simulink model "TVModel"  (R2022a)
settings: Solver=FixedStepDiscrete  StartTime=0.0  StopTime=10.0  FixedStep=0.02  MaxStep=0.01  RelTol=1e-3
undefined symbols (not defined in the file or in its folder): MB, TV, TV_OLD
libraries: simulink x22, simulink_extras x14, slpidlib x8, fuzblock x5, controlLib x4, dspstat3 x4, eeGeneralControl x3, cstblocks x3, eeSlidingModeController x1, sharedTrackingLibrary x1
(part 8 of 8)

== stateflow chart TVModel/Subsystem/Subsystem1/Torque Distribution/MPC/Faults Detection/Overlap Chart ==
  state Stop
    en:
    torque_flag = 0;
  state Go
    en:
    torque_flag = 1;
  (default) -> Go
  Go -> Stop : [brake > 0]
  Stop -> Go : [(brake<=0.05 && throttle<0.05)]
  data: throttle input; brake input; torque_flag output

== matlab function TVModel/Subsystem/Subsystem1/Torque Distribution/MPC/Mz Generation/MATLAB Function2 ==
  data: Nhorizon input; vx input; vy input; Nx output; YRD input; r input; delta input; ax input; ay input; kappa input
function Nx =fcn(Nhorizon,vx,vy,YRD,r,delta,ax,ay,kappa)

g   = 9.81;            % [m/s^2]                          
wd  = 0.48;             % [~]         
wb  = 1.53;            % [~]          
tf  = 1.27;            % [m]          
tr  = 1.27;            % [m]          
m   = 195+75;          % [Kg]            
Iz  = 180;             % [Kg*m^2]      % 227    
a   = wb*wd;           % [m]            
b   = wb - a;          % [m]            
hcog = 0.29;           % [m]           
Fzf  = m*g/2*(wd);     % [N]                 
Fzr  = m*g/2*(1-wd);   % [N]                   
tau = 13.5;            % [~]          
rs  = 0.235;           % [m]     
LMU = 0.8;
dt = 0.02;

% ~~~~~~~~~~~~~~~~~~~~~~~~~~~ Aero parameters ~~~~~~~~~~~~~~~~~~~~~~~~~~~~~
xcop = 0.6810;
hcop = 0.576;          % [m]      
rho = 1.225;           % [Kg/m^3]     
CdA = 1.708;           % [m]     
ClA = 5.14;            % [m]   

kappa_FL = kappa(1);
kappa_FR = kappa(2);
kappa_RL = kappa(3);
kappa_RR = kappa(4);

% ~~~~~~~~~~~~~~~~~~~~~~~~~~~ Aerodynamics ~~~~~~~~~~~~~~~~~~~~~~~~~~~~~~~~
Faerox = 0.5*rho*CdA*vx^2;
Faeroz = 0.5*rho*ClA*vx^2;

% ~~~~~~~~~~~~~~~~~~~~~~~~~~~ Slip Angles ~~~~~~~~~~~~~~~~~~~~~~~~~~~~~~~~~
alpha_FL =  (atan((vy + r*a)./(vx - r*tf/2)) - delta);
alpha_FR =  (atan((vy + r*a)./(vx + r*tf/2)) - delta);
alpha_RL =  (atan((vy - r*b)./(vx - r*tr/2)));     
alpha_RR =  (atan((vy - r*b)./(vx + r*tr/2)));     

% ~~~~~~~~~~~~~~~~~~~~~~~~~~~ Vertical loads ~~~~~~~~~~~~~~~~~~~~~~~~~~~~~~

Fz_FL = Fzf - 0.5*(m/tf*hcog).*ay + 0.5*Faeroz*(1-xcop/wb) - 0.5*Faerox/wb*hcop - 0.5*(m/wb*hcog).*ax;
Fz_FR = Fzf + 0.5*(m/tf*hcog).*ay + 0.5*Faeroz*(1-xcop/wb) - 0.5*Faerox/wb*hcop - 0.5*(m/wb*hcog).*ax;
Fz_RL = Fzr - 0.5*(m/tr*hcog).*ay + 0.5*Faeroz*(xcop/wb) + 0.5*Faerox/wb*hcop + 0.5*(m/wb*hcog).*ax;
Fz_RR = Fzr + 0.5*(m/tr*hcog).*ay + 0.5*Faeroz*(xcop/wb) + 0.5*Faerox/wb*hcop + 0.5*(m/wb*hcog).*ax;

% ~~~~~~~~~~~~~~~~~~~~~~~~ Camber gain with steer ~~~~~~~~~~~~~~~~~~~~~~~~~
% ~~~~~~~~~~~~~~~~~~~~~~~~~~ Lateral forces ~~~~~~~~~~~~~~~~~~~~~~~~~~~~~~~
Fy_FL = tire_model(Fz_FL,kappa_FL,alpha_FL,0,LMU);
Fy_FR = tire_model(Fz_FR,kappa_FR,alpha_FR,0,LMU);
Fy_RL = tire_model(Fz_RL,kappa_RL,alpha_RL,0,LMU);
Fy_RR = tire_model(Fz_RR,kappa_RR,alpha_RR,0,LMU);

% ~~~~~~~~~~~~~~~~~~~~~~~~~~~ E.o.M. Balance ~~~~~~~~~~~~~~~~~~~~~~~~~~~~~~
Ny = (Fy_FL + Fy_FR).*cos(delta).*a - b*(Fy_RL + Fy_RR) + tf*(- (Fy_FR - Fy_FL).*sin(delta))/2;
% ~~~~~~~~~~~~~~~~~~~~~~~~~~~ System Dynamics f(x,u) ~~~~~~~~~~~~~~~~~~~~~~     
Nx = (YRD-r)/(dt*Nhorizon)*Iz - Ny;

if(isnan(Nx))
    Nx = 0;
end
end
%% ~~~~~~~~~~~~~~~~~~~~~~~~~~ Functions ~~~~~~~~~~~~~~~~~~~~~~~~~~~~~~~~~~~
function y = tire_model(Fz,kappa,alpha,gamma,LMU)
% Old tir file
% y = - (1.0*cos(0.958*atan((13.9*(3.86e-7*Fz - 1.0*kappa + 2.05e-4))/((12.4*alpha - 0.512)^2 + 1.0)^(1/2) + (atan((13.9*(3.86e-7*Fz - 1.0*kappa + 2.05e-4))/((12.4*alpha - 0.512)^2 + 1.0)^(1/2)) - (13.9*(3.86e-7*Fz - 1.0*kappa + 2.05e-4))/((12.4*alpha - 0.512)^2 + 1.0)^(1/2))*(0.0013*Fz - 2.33)))*(Fz*LMU*(2.59e-6*Fz + 0.0594) - 1.0*Fz*LMU*sin(1.1*atan((1.18*sign(3.32e-6*Fz - 1.0*alpha + 2.0e-5) + 1.0)*(atan((3.41e+4*sin(2.0*atan(8.72e-4*Fz))*(3.32e-6*Fz - 1.0*alpha + 2.0e-5))/(1.1*Fz*LMU*(4.11e-4*Fz - 2.12) - 0.01)) - (3.41e+4*sin(2.0*atan(8.72e-4*Fz))*(3.32e-6*Fz - 1.0*alpha + 2.0e-5))/(1.1*Fz*LMU*(4.11e-4*Fz - 2.12) - 0.01))*(6.75e-4*Fz - 0.451) + (3.41e+4*sin(2.0*atan(8.72e-4*Fz))*(3.32e-6*Fz - 1.0*alpha + 2.0e-5))/(1.1*Fz*LMU*(4.11e-4*Fz - 2.12) - 0.01)))*(4.11e-4*Fz - 2.12)))/cos(0.958*atan((atan((13.9*(3.86e-7*Fz + 2.05e-4))/((12.4*alpha - 0.512)^2 + 1.0)^(1/2)) - (13.9*(3.86e-7*Fz + 2.05e-4))/((12.4*alpha - 0.512)^2 + 1.0)^(1/2))*(0.0013*Fz - 2.33) + (13.9*(3.86e-7*Fz + 2.05e-4))/((12.4*alpha - 0.512)^2 + 1.0)^(1/2))) - (1.0*Fz*LMU*sin(1.94*atan(16.1*kappa))*(1.03e-5*Fz - 2.88e-4)*(4.11e-4*Fz - 2.12))/(225.0*alpha^2 + 1.0)^(1/2);
% New tir file
y = (cos(0.958*atan((13.9*(3.86e-7*Fz - 1.0*kappa + 2.05e-4))/((12.4*alpha - 0.512)^2 + 1.0)^(1/2) + (atan((13.9*(3.86e-7*Fz - 1.0*kappa + 2.05e-4))/((12.4*alpha - 0.512)^2 + 1.0)^(1/2)) - (13.9*(3.86e-7*Fz - 1.0*kappa + 2.05e-4))/((12.4*alpha - 0.512)^2 + 1.0)^(1/2))*(0.0013*Fz - 2.33)))*(Fz*LMU*(7.1e-5*Fz - 0.149) + Fz*LMU*sin(1.34*atan((3.45e+4*sin(2.0*atan(5.59e-4*Fz))*(1.14e-6*Fz - 1.0*alpha + 0.00239))/(1.34*Fz*LMU*(2.82e-4*Fz - 2.02) - 0.01) - 1.0*(0.26*sign(1.14e-6*Fz - 1.0*alpha + 0.00239) + 1.0)*(3.99e-5*Fz - 0.521)*(atan((3.45e+4*sin(2.0*atan(5.59e-4*Fz))*(1.14e-6*Fz - 1.0*alpha + 0.00239))/(1.34*Fz*LMU*(2.82e-4*Fz - 2.02) - 0.01)) - (3.45e+4*sin(2.0*atan(5.59e-4*Fz))*(1.14e-6*Fz - 1.0*alpha + 0.00239))/(1.34*Fz*LMU*(2.82e-4*Fz - 2.02) - 0.01))))*(2.82e-4*Fz - 2.02)))/cos(0.958*atan((atan((13.9*(3.86e-7*Fz + 2.05e-4))/((12.4*alpha - 0.512)^2 + 1.0)^(1/2)) - (13.9*(3.86e-7*Fz + 2.05e-4))/((12.4*alpha - 0.512)^2 + 1.0)^(1/2))*(0.0013*Fz - 2.33) + (13.9*(3.86e-7*Fz + 2.05e-4))/((12.4*alpha - 0.512)^2 + 1.0)^(1/2))) - (1.0*Fz*LMU*sin(1.94*atan(16.1*kappa))*(2.82e-4*Fz - 2.02)*(1.03e-5*Fz - 2.88e-4))/(225.0*alpha^2 + 1.0)^(1/2);
end

== matlab function TVModel/Subsystem/Subsystem1/Torque Distribution/MPC/States Constraints/Cross Check ==
  data: ubx_in input; bounds input; ubx_out output; lbx_in input; lbx_out output; epsilon input; throttle input; brake input
function [ubx_out,lbx_out] = fcn(ubx_in,bounds,lbx_in,epsilon,throttle,brake)
    
    ubx_out = ubx_in;
    lbx_out = lbx_in;
    lbx_max = bounds(10);
    
    % cross between bounds
    switch epsilon
        case 1
            for i = 1 : 4
                if lbx_in(i) > ubx_in(i)
                   lbx_out(i) = ubx_in(i) - lbx_max;
                end
            end
        case 0
            if throttle > 0.05
               for i = 1 : 4
                   lbx_out(i) = 0;
               end
            elseif brake > 0.05
               for i = 1 : 4
                   ubx_out(i) = 0;
               end       
            else
            end
    end
end

== matlab function TVModel/Subsystem/Subsystem1/Torque Distribution/MPC/Polytropic Matrix/MATLAB Function ==
  data: y output; Limit input; delta input
function y = fcn(Limit,delta)

tf = 1.27;
tr = 1.27;
a = 0.765;

delta_l = delta(1);
delta_r = delta(2);

% C = zeros(5,7);

C = [0 , 0 , 0 , 1 , 1 , 1 , 1;
     0 , 0 , 0 , Limit(1)/1000 , Limit(2)/1000 , Limit(3)/1000 , Limit(4)/1000;
     0 , 0 , 0 , 0 , 1 , 0 ,-1;
     0 , 0 , 0 , 1 , 0 ,-1 , 0;
     0 , 0 , 0 ,+a.*sin(delta_l)-tf/2.*cos(delta_l),+a.*sin(delta_r)+tf/2*cos(delta_r),-tr/2,tr/2];

y = C(:);

== matlab function TVModel/Subsystem/Subsystem1/Torque Distribution/MPC/Weights Generation/Efficiency limit/MATLAB Function ==
  data: u input; u output; T input
function u = fcn(u,T)

for i = 1 : 4
    if T(i) <= 0 
       u(i) = 0; 
    end
end

== matlab function TVModel/Subsystem/Subsystem1/Torque Distribution/MPC/Weights Generation/MATLAB Function ==
  data: u input; y output; deltaAxle input
function y = fcn(u,deltaAxle)

Q = diag([u(1),u(2),u(3),u(4),u(5),u(6),u(7)]);
R = diag([u(8),u(9),u(10),u(11)]);
unscale = 50;
W = blkdiag(Q, R);

W(4,6) = -deltaAxle;
W(6,4) = W(4,6);

W(5,7) = -deltaAxle;
W(7,5) = W(5,7);

W = unscale*W;

y = W(:);

== matlab function TVModel/Subsystem/Subsystem1/Torque Distribution/Reference Tracking/MATLAB Function ==
  data: LUT_brk input; brk input; YRD output; LUT_thr input
function YRD = fcn(LUT_brk,brk,LUT_thr)

YRD = LUT_brk*brk + LUT_thr*(1 - brk) ;

== matlab function TVModel/Subsystem/Subsystem1/Torque Distribution/MPC/USEFUL STUFFFF/Subsystem/MATLAB Function ==
  data: T input; Tnew output; Plim input; Eta input; Omega input; Torque input; Omega_motors input; k output; fx output; brake_flag input
function [Tnew,k,fx] = fcn(T,Plim,Eta,Omega,Torque,Omega_motors,brake_flag)

Tnew = zeros(4,1);
fx = 10^3;
k      = 0;

exit   = 0;
dT     = 0;
eps    = 0.01;
h      = 0.3;
dT_new = 0;

eta_Plim = 1;

while exit == 0

    if brake_flag == 0;
        Tnew(1) = T(1) - dT;
        Tnew(2) = T(2) - dT;
        Tnew(3) = T(3) - dT;
        Tnew(4) = T(4) - dT;  
    
        eta = efficiency(Eta,Omega,Torque,Tnew,Omega_motors);
   

        for i = 1 : 4
            if Tnew(i) <= 0 
               Tnew(i) = 0;
            end
        end
    else
        Tnew(1) = T(1) + dT;
        Tnew(2) = T(2) + dT;
        Tnew(3) = T(3) + dT;
        Tnew(4) = T(4) + dT;  
    
        eta = efficiency(Eta,Omega,Torque,Tnew,Omega_motors);
   

        for i = 1 : 4
            if Tnew(i) >= 0 
               Tnew(i) = 0;
            end
        end
    end
%     eta1_hplus = efficiency(Eta,Omega,Torque,T1 - (dT + h),w1);
%     eta1_hminus = efficiency(Eta,Omega,Torque,T1 - (dT -h),w1);
%     eta2_hplus = efficiency(Eta,Omega,Torque,T2 - (dT + h),w2);
%     eta2_hminus = efficiency(Eta,Omega,Torque,T2 - (dT -h),w2);  
    fx = ( dot(Tnew./eta,Omega_motors') - Plim*eta_Plim );
    dT_new = dT + h;
    
%     fdotx = (-1/eta1/ ((eta1_hplus - eta1_hminus)/(2*h)) -1/eta2/ ((eta2_hplus - eta2_hminus)/(2*h)) );
%     dT_new = dT -  fx/fdotx;
    if k >= 100 || fx<0 || isnan(fx)
       exit = 1;
    else 
       dT = dT_new;
       k = k + 1;
    end

end

end

function eta = efficiency(Eta,Omega,Torque,T,w)    
         eta = interp2(Torque,Omega,Eta,abs(T),abs(w),"linear");
end

== stateflow chart TVModel/Subsystem/Subsystem1/Torque Limits/Torque Request/T_Req_Chart ==
  state Brake
    en:
    t_req=1;
  state Throttle
    en:
    t_req=0;
  (default) -> Throttle
  Brake -> Throttle : [brake<=0 && throttle<0.05]
  Throttle -> Brake : [brake>0]
  data: brake input; throttle input; t_req output

== matlab function TVModel/Subsystem/Subsystem1/Torque Distribution/MPC/Faults Detection/Simple torque/No_TV/MATLAB Function ==
  data: T input; Tnew output; Plim input; Eta input; Omega input; Torque input; Omega_motors input; k output; fx output; brake_flag input
function [Tnew,k,fx] = fcn(T,Plim,Eta,Omega,Torque,Omega_motors,brake_flag)

Tnew = zeros(4,1);
fx = 10^3;
k      = 0;

exit   = 0;
dT     = 0;
eps    = 0.01;
h      = 0.3;
dT_new = 0;

eta_Plim = 1;

while exit == 0

    if brake_flag == 0;
        Tnew(1) = T(1) - dT;
        Tnew(2) = T(2) - dT;
        Tnew(3) = T(3) - dT;
        Tnew(4) = T(4) - dT;  
    
        eta = efficiency(Eta,Omega,Torque,Tnew,Omega_motors);
   

        for i = 1 : 4
            if Tnew(i) <= 0 
               Tnew(i) = 0;
            end
        end
    else
        Tnew(1) = T(1) + dT;
        Tnew(2) = T(2) + dT;
        Tnew(3) = T(3) + dT;
        Tnew(4) = T(4) + dT;  
    
        eta = efficiency(Eta,Omega,Torque,Tnew,Omega_motors);
   

        for i = 1 : 4
            if Tnew(i) >= 0 
               Tnew(i) = 0;
            end
        end
    end
%     eta1_hplus = efficiency(Eta,Omega,Torque,T1 - (dT + h),w1);
%     eta1_hminus = efficiency(Eta,Omega,Torque,T1 - (dT -h),w1);
%     eta2_hplus = efficiency(Eta,Omega,Torque,T2 - (dT + h),w2);
%     eta2_hminus = efficiency(Eta,Omega,Torque,T2 - (dT -h),w2);  
    fx = ( dot(Tnew./eta,Omega_motors') - Plim*eta_Plim );
    dT_new = dT + h;
    
%     fdotx = (-1/eta1/ ((eta1_hplus - eta1_hminus)/(2*h)) -1/eta2/ ((eta2_hplus - eta2_hminus)/(2*h)) );
%     dT_new = dT -  fx/fdotx;
    if k >= 100 || fx<0 || isnan(fx)
       exit = 1;
    else 
       dT = dT_new;
       k = k + 1;
    end

end

end

function eta = efficiency(Eta,Omega,Torque,T,w)    
         eta = interp2(Torque,Omega,Eta,abs(T),abs(w),"linear");
end

== matlab function TVModel/Subsystem/Subsystem1/Torque Distribution/MPC/Useful Calculations/MATLAB Function ==
  data: T input; y output; delta input
function y = fcn(T,delta)

tf = 1.27;
tr = 1.27;
a = 0.765;

delta_l = delta(1);
delta_r = delta(2);

y = sum(T.*[a.*sin(delta_l)-tf/2.*cos(delta_l);+a.*sin(delta_r)+tf/2*cos(delta_r);-tr/2;tr/2]);

== stateflow chart TVModel/Subsystem/Subsystem1/Torque Distribution/MPC/Mz Generation/Chart ==
  state OFF
    en,du:
    mz_output = 0;
  state ON
    en,du:
    mz_output = mz_controller;
  state SWITCHING_FILTER
    en,du:
    mz_output = mz_filter_tau*mz_output;
  (default) -> OFF
  OFF -> ON : [epsilon == 1]
  SWITCHING_FILTER -> ON [order 2] : [ epsilon == 1]
  SWITCHING_FILTER -> OFF [order 1] : [count(in(SWITCHING_FILTER)) > mz_filter_time/ts]
  ON -> SWITCHING_FILTER : [epsilon == 0]
  data: mz_controller input; mz_output output; ts constant double =TV.MPC.T; mz_filter_time constant double =TV.MPC.mz_filter_time; mz_filter_tau constant double =TV.MPC.mz_filter_tau; epsilon input

== matlab function TVModel/Subsystem/Subsystem1/Slip Control/Traction Control/Subsystem/Mu Linearization ==
  data: kappa input; mu0 output; mu1 output; Fz input; a0 output
function [mu0,mu1,a0] = fcn(kappa,Fz)

LMUX = 0.93;
J_wheel = 2e5/1e6;
rs = 0.235;
m = 270/4;
tau = 13.5;
dt = 0.02;

deltaKappa = 0.01;
kappa_plus = kappa + deltaKappa;

mu0 = muX(kappa,Fz,LMUX);
mu1 = (muX(kappa_plus,Fz,LMUX)-mu0)./(deltaKappa);

a0 = Fz./vx*mu1( (1-kappa)/m + rs^2/J_wheel );

end
function mu = muX(kappa,Fz,LMUX)
    mu = ((Fz.^2.*LMUX)./1.0e+4-Fz.*LMUX.*sin(atan((Fz.*5.946e-5-6.5736e-1).*(sign(Fz.*(-1.5696e-6)+kappa+6.665e-4).*5.242e-1+1.0).*(atan((Fz.*exp(Fz.*(-1.3455e-5)+1.3455e-2).*(Fz.*(3.0./2.0e+2)+6.77e+2./1.0e+1).*(Fz.*(-1.5696e-6)+kappa+6.665e-4).*(3.33e+2./4.0e+2))./(Fz.*LMUX.*2.5847808+1.0./1.0e+2))-(Fz.*exp(Fz.*(-1.3455e-5)+1.3455e-2).*(Fz.*(3.0./2.0e+2)+6.77e+2./1.0e+1).*(Fz.*(-1.5696e-6)+kappa+6.665e-4).*(3.33e+2./4.0e+2))./(Fz.*LMUX.*2.5847808+1.0./1.0e+2))-(Fz.*exp(Fz.*(-1.3455e-5)+1.3455e-2).*(Fz.*(3.0./2.0e+2)+6.77e+2./1.0e+1).*(Fz.*(-1.5696e-6)+kappa+6.665e-4).*(3.33e+2./4.0e+2))./(Fz.*LMUX.*2.5847808+1.0./1.0e+2)).*(1.68e+2./1.25e+2)).*1.9232)./Fz;
end

== stateflow chart TVModel/Subsystem/Subsystem1/Slip Control/Traction Control/Subsystem/Subsystem/Chart ==
  state OFF
    en,du:
    TC_max = [21];
  state ON
    en,du:
    TC_max = T_ff ;
  state SWITCHING_FILTER
    en,du:
    TC_max = TC_filter_tau*TC_max;
  (default) -> OFF
  OFF -> ON : [epsilon == 1]
  SWITCHING_FILTER -> ON [order 2] : [ epsilon == 1]
  SWITCHING_FILTER -> OFF [order 1] : [count(in(SWITCHING_FILTER)) > TC_filter_time/ts]
  ON -> SWITCHING_FILTER : [epsilon == 0]
  data: T_ff input; TC_max output; ts constant double =TV.MPC.T; TC_filter_time constant double =TV.MPC.mz_filter_time; TC_filter_tau constant double =TV.MPC.mz_filter_tau; epsilon input

== stateflow chart TVModel/Subsystem/Subsystem1/Slip Control/Traction Control/Subsystem/Subsystem/Chart1 ==
  state OFF
    en,du:
    TC_max = [21];
  state ON
    en,du:
    TC_max = T_ff ;
  state SWITCHING_FILTER
    en,du:
    TC_max = TC_filter_tau*TC_max;
  (default) -> OFF
  OFF -> ON : [epsilon == 1]
  SWITCHING_FILTER -> ON [order 2] : [ epsilon == 1]
  SWITCHING_FILTER -> OFF [order 1] : [count(in(SWITCHING_FILTER)) > TC_filter_time/ts]
  ON -> SWITCHING_FILTER : [epsilon == 0]
  data: T_ff input; TC_max output; ts constant double =TV.MPC.T; TC_filter_time constant double =TV.MPC.mz_filter_time; TC_filter_tau constant double =TV.MPC.mz_filter_tau; epsilon input

== stateflow chart TVModel/Subsystem/Subsystem1/Slip Control/Traction Control/Subsystem/Subsystem/Chart2 ==
  state OFF
    en,du:
    TC_max = [21];
  state ON
    en,du:
    TC_max = T_ff ;
  state SWITCHING_FILTER
    en,du:
    TC_max = TC_filter_tau*TC_max;
  (default) -> OFF
  OFF -> ON : [epsilon == 1]
  SWITCHING_FILTER -> ON [order 2] : [ epsilon == 1]
  SWITCHING_FILTER -> OFF [order 1] : [count(in(SWITCHING_FILTER)) > TC_filter_time/ts]
  ON -> SWITCHING_FILTER : [epsilon == 0]
  data: T_ff input; TC_max output; ts constant double =TV.MPC.T; TC_filter_time constant double =TV.MPC.mz_filter_time; TC_filter_tau constant double =TV.MPC.mz_filter_tau; epsilon input

== stateflow chart TVModel/Subsystem/Subsystem1/Slip Control/Traction Control/Subsystem/Subsystem/Chart3 ==
  state OFF
    en,du:
    TC_max = [21];
  state ON
    en,du:
    TC_max = T_ff ;
  state SWITCHING_FILTER
    en,du:
    TC_max = TC_filter_tau*TC_max;
  (default) -> OFF
  OFF -> ON : [epsilon == 1]
  SWITCHING_FILTER -> ON [order 2] : [ epsilon == 1]
  SWITCHING_FILTER -> OFF [order 1] : [count(in(SWITCHING_FILTER)) > TC_filter_time/ts]
  ON -> SWITCHING_FILTER : [epsilon == 0]
  data: T_ff input; TC_max output; ts constant double =TV.MPC.T; TC_filter_time constant double =TV.MPC.mz_filter_time; TC_filter_tau constant double =TV.MPC.mz_filter_tau; epsilon input

== matlab function TVModel/Subsystem/Subsystem1/Slip Control/Traction Control/Subsystem1/MATLAB Function1 ==
  data: vx input; T_ff output; kappa input; Fz input; kappa_p input; omega_p input; T_ff_deceleration output; T_ff_slip output
function [T_ff,T_ff_deceleration,T_ff_slip] = fcn(vx,kappa,Fz,kappa_p,omega_p)

LMU = 0.93;
J_wheel = 2e5/1e6;
rs = 0.235;
m = 270/4;
tau = 13.5;
dt = 0.02;
g = 9.81;

% @(Fz,LMUX,kappa)
% Old tire
% muX = ((Fz.^2.*LMUX)./1.0e+4-Fz.*LMUX.*sin(atan((Fz.*5.946e-5-6.5736e-1).*(sign(Fz.*(-1.5696e-6)+kappa+6.665e-4).*5.242e-1+1.0).*(atan((Fz.*exp(Fz.*(-1.3455e-5)+1.3455e-2).*(Fz.*(3.0./2.0e+2)+6.77e+2./1.0e+1).*(Fz.*(-1.5696e-6)+kappa+6.665e-4).*(3.33e+2./4.0e+2))./(Fz.*LMUX.*2.5847808+1.0./1.0e+2))-(Fz.*exp(Fz.*(-1.3455e-5)+1.3455e-2).*(Fz.*(3.0./2.0e+2)+6.77e+2./1.0e+1).*(Fz.*(-1.5696e-6)+kappa+6.665e-4).*(3.33e+2./4.0e+2))./(Fz.*LMUX.*2.5847808+1.0./1.0e+2))-(Fz.*exp(Fz.*(-1.3455e-5)+1.3455e-2).*(Fz.*(3.0./2.0e+2)+6.77e+2./1.0e+1).*(Fz.*(-1.5696e-6)+kappa+6.665e-4).*(3.33e+2./4.0e+2))./(Fz.*LMUX.*2.5847808+1.0./1.0e+2)).*(1.68e+2./1.25e+2)).*1.9232)./Fz;

% New tire
muX = (1.0e-4.*Fz.^2.*LMU - 1.92.*Fz.*LMU.*sin(1.41.*atan(0.7.*(5.95e-5.*Fz - 0.657).*(0.524*sign(kappa - 1.57e-6.*Fz + 6.66e-4) + 1.0).*(atan((0.7.*Fz.*exp(0.0135 - 1.35e-5.*Fz).*(0.015.*Fz + 67.7).*(kappa - 1.57e-6.*Fz + 6.66e-4))./(2.71.*Fz.*LMU + 0.01)) - (0.7.*Fz.*exp(0.0135 - 1.35e-5.*Fz).*(0.015.*Fz + 67.7).*(kappa - 1.57e-6.*Fz + 6.66e-4))./(2.71.*Fz.*LMU + 0.01)) - (0.7.*Fz.*exp(0.0135 - 1.35e-5.*Fz).*(0.015.*Fz + 67.7).*(kappa - 1.57e-6.*Fz + 6.66e-4))./(2.71.*Fz.*LMU + 0.01))))./Fz;

T_ff_slip = (kappa_p + 1/vx.*( (1-kappa)/m + rs^2/J_wheel ).*Fz.*muX).*vx.*J_wheel/rs/tau;

eta = - omega_p*rs/g;

T_ff_deceleration = (+rs.^2./J_wheel./g.*muX.*Fz - eta).*J_wheel.*g/rs/tau/2;

% alpha = 0.96;
alpha = 1;

T_ff = T_ff_slip*alpha + T_ff_deceleration*(1 - alpha);

end

== matlab function TVModel/Subsystem/Subsystem1/Slip Control/Traction Control/Subsystem1/Mu Linearization ==
  data: kappa input; mu0 output; mu1 output; Fz input; a0 output
function [mu0,mu1,a0] = fcn(kappa,Fz)

LMUX = 0.93;
J_wheel = 2e5/1e6;
rs = 0.235;
m = 270/4;
tau = 13.5;
dt = 0.02;

deltaKappa = 0.01;
kappa_plus = kappa + deltaKappa;

mu0 = muX(kappa,Fz,LMUX);
mu1 = (muX(kappa_plus,Fz,LMUX)-mu0)./(deltaKappa);

a0 = Fz./vx*mu1( (1-kappa)/m + rs^2/J_wheel );

end
function mu = muX(kappa,Fz,LMUX)
    mu = ((Fz.^2.*LMUX)./1.0e+4-Fz.*LMUX.*sin(atan((Fz.*5.946e-5-6.5736e-1).*(sign(Fz.*(-1.5696e-6)+kappa+6.665e-4).*5.242e-1+1.0).*(atan((Fz.*exp(Fz.*(-1.3455e-5)+1.3455e-2).*(Fz.*(3.0./2.0e+2)+6.77e+2./1.0e+1).*(Fz.*(-1.5696e-6)+kappa+6.665e-4).*(3.33e+2./4.0e+2))./(Fz.*LMUX.*2.5847808+1.0./1.0e+2))-(Fz.*exp(Fz.*(-1.3455e-5)+1.3455e-2).*(Fz.*(3.0./2.0e+2)+6.77e+2./1.0e+1).*(Fz.*(-1.5696e-6)+kappa+6.665e-4).*(3.33e+2./4.0e+2))./(Fz.*LMUX.*2.5847808+1.0./1.0e+2))-(Fz.*exp(Fz.*(-1.3455e-5)+1.3455e-2).*(Fz.*(3.0./2.0e+2)+6.77e+2./1.0e+1).*(Fz.*(-1.5696e-6)+kappa+6.665e-4).*(3.33e+2./4.0e+2))./(Fz.*LMUX.*2.5847808+1.0./1.0e+2)).*(1.68e+2./1.25e+2)).*1.9232)./Fz;
end

== stateflow chart TVModel/Subsystem/Subsystem1/Slip Control/Traction Control/Subsystem1/Subsystem/Chart ==
  state OFF
    en,du:
    TC_max = [21];
  state ON
    en,du:
    TC_max = T_ff ;
  state SWITCHING_FILTER
    en,du:
    TC_max = TC_filter_tau*TC_max;
  (default) -> OFF
  OFF -> ON : [epsilon == 1]
  SWITCHING_FILTER -> ON [order 2] : [ epsilon == 1]
  SWITCHING_FILTER -> OFF [order 1] : [count(in(SWITCHING_FILTER)) > TC_filter_time/ts]
  ON -> SWITCHING_FILTER : [epsilon == 0]
  data: T_ff input; TC_max output; ts constant double =TV.MPC.T; TC_filter_time constant double =TV.MPC.mz_filter_time; TC_filter_tau constant double =TV.MPC.mz_filter_tau; epsilon input

== stateflow chart TVModel/Subsystem/Subsystem1/Slip Control/Traction Control/Subsystem1/Subsystem/Chart1 ==
  state OFF
    en,du:
    TC_max = [21];
  state ON
    en,du:
    TC_max = T_ff ;
  state SWITCHING_FILTER
    en,du:
    TC_max = TC_filter_tau*TC_max;
  (default) -> OFF
  OFF -> ON : [epsilon == 1]
  SWITCHING_FILTER -> ON [order 2] : [ epsilon == 1]
  SWITCHING_FILTER -> OFF [order 1] : [count(in(SWITCHING_FILTER)) > TC_filter_time/ts]
  ON -> SWITCHING_FILTER : [epsilon == 0]
  data: T_ff input; TC_max output; ts constant double =TV.MPC.T; TC_filter_time constant double =TV.MPC.mz_filter_time; TC_filter_tau constant double =TV.MPC.mz_filter_tau; epsilon input

== stateflow chart TVModel/Subsystem/Subsystem1/Slip Control/Traction Control/Subsystem1/Subsystem/Chart2 ==
  state OFF
    en,du:
    TC_max = [21];
  state ON
    en,du:
    TC_max = T_ff ;
  state SWITCHING_FILTER
    en,du:
    TC_max = TC_filter_tau*TC_max;
  (default) -> OFF
  OFF -> ON : [epsilon == 1]
  SWITCHING_FILTER -> ON [order 2] : [ epsilon == 1]
  SWITCHING_FILTER -> OFF [order 1] : [count(in(SWITCHING_FILTER)) > TC_filter_time/ts]
  ON -> SWITCHING_FILTER : [epsilon == 0]
  data: T_ff input; TC_max output; ts constant double =TV.MPC.T; TC_filter_time constant double =TV.MPC.mz_filter_time; TC_filter_tau constant double =TV.MPC.mz_filter_tau; epsilon input

== stateflow chart TVModel/Subsystem/Subsystem1/Slip Control/Traction Control/Subsystem1/Subsystem/Chart3 ==
  state OFF
    en,du:
    TC_max = [21];
  state ON
    en,du:
    TC_max = T_ff ;
  state SWITCHING_FILTER
    en,du:
    TC_max = TC_filter_tau*TC_max;
  (default) -> OFF
  OFF -> ON : [epsilon == 1]
  SWITCHING_FILTER -> ON [order 2] : [ epsilon == 1]
  SWITCHING_FILTER -> OFF [order 1] : [count(in(SWITCHING_FILTER)) > TC_filter_time/ts]
  ON -> SWITCHING_FILTER : [epsilon == 0]
  data: T_ff input; TC_max output; ts constant double =TV.MPC.T; TC_filter_time constant double =TV.MPC.mz_filter_time; TC_filter_tau constant double =TV.MPC.mz_filter_tau; epsilon input

== stateflow chart TVModel/Subsystem/Subsystem1/Slip Control/Traction Control/Slip Control/ABS/Activation logic ==
  state TS_ON
    state ABS_OFF
      en,du:
      T_min(1:4) = -T_limit(1:4);
    state ABS_ON
      state FL [parallel]
        settings: executionOrder=1
        state ABS_ACTIVE
          en:
          T_min(1) = T_actual(1);
          du:
          T_min(1) = Tmin_PI(1);
        state ABS_INACTIVE
          en,du:
          T_min(1) = -T_limit(1);
        (default) -> TS_ON.ABS_ON.FL.ABS_INACTIVE
        TS_ON.ABS_ON.FL.ABS_INACTIVE -> TS_ON.ABS_ON.FL.ABS_ACTIVE : [eps(1) <= (epsTarget(1) - slipNoise) && T_actual(1)<0]
        TS_ON.ABS_ON.FL.ABS_ACTIVE -> TS_ON.ABS_ON.FL.ABS_INACTIVE : [T_actual(1) > slipDeactPerc*Tmin_old(1)]
      state FR [parallel]
        settings: executionOrder=2
        state ABS_ACTIVE
          en:
          T_min(2) = T_actual(2);
          du:
          T_min(2) = Tmin_PI(2);
        state ABS_INACTIVE
          en,du:
          T_min(2) = -T_limit(2);
        (default) -> TS_ON.ABS_ON.FR.ABS_INACTIVE
        TS_ON.ABS_ON.FR.ABS_INACTIVE -> TS_ON.ABS_ON.FR.ABS_ACTIVE : [eps(2) <= (epsTarget(2) - slipNoise) && T_actual(2)<0]
        TS_ON.ABS_ON.FR.ABS_ACTIVE -> TS_ON.ABS_ON.FR.ABS_INACTIVE : [T_actual(2) > slipDeactPerc*Tmin_old(2) ]
      state RL [parallel]
        settings: executionOrder=3
        state ABS_ACTIVE
          en:
          T_min(3) = T_actual(3);
          du:
          T_min(3) = Tmin_PI(3);
        state ABS_INACTIVE
          en,du:
          T_min(3) = -T_limit(3);
        (default) -> TS_ON.ABS_ON.RL.ABS_INACTIVE
        TS_ON.ABS_ON.RL.ABS_INACTIVE -> TS_ON.ABS_ON.RL.ABS_ACTIVE : [eps(3) <= (epsTarget(3) - slipNoise) && T_actual(3)<0]
        TS_ON.ABS_ON.RL.ABS_ACTIVE -> TS_ON.ABS_ON.RL.ABS_INACTIVE : [T_actual(3) > slipDeactPerc*Tmin_old(3)]
      state RR [parallel]
        settings: executionOrder=4
        state ABS_ACTIVE
          en:
          T_min(4) = T_actual(4);
          du:
          T_min(4) = Tmin_PI(4);
        state ABS_INACTIVE
          en,du:
          T_min(4) = -T_limit(4);
        (default) -> TS_ON.ABS_ON.RR.ABS_INACTIVE
        TS_ON.ABS_ON.RR.ABS_INACTIVE -> TS_ON.ABS_ON.RR.ABS_ACTIVE : [eps(4) <= (epsTarget(4) - slipNoise) && T_actual(4)<0]
        TS_ON.ABS_ON.RR.ABS_ACTIVE -> TS_ON.ABS_ON.RR.ABS_INACTIVE : [T_actual(4) > slipDeactPerc*Tmin_old(4)]
    (default) -> ABS_OFF
    ABS_ON -> ABS_OFF : [TC_flag == 0]
    ABS_OFF -> ABS_ON : [TC_flag == 1]
  state TS_OFF
    en:
    T_min(1:4) =zeros(4,1);
  (default) -> TS_OFF
  TS_OFF -> TS_ON : [RTD_flag == 1]
  TS_ON -> TS_OFF : [RTD_flag == 0]
  data: Tmin_PI input size=4; epsTarget input size=4; eps input size=4; T_actual input size=4 =zeros(4,1); T_min output size=4 =zeros(4,1); T_limit input size=4; TC_flag input size=1; Tmin_old input size=4; slipNoise input double =LV.SLIP.; slipDeactPerc input; RTD_flag input

== matlab function TVModel/Subsystem/Subsystem1/Slip Control/Traction Control/Slip Control/Slip computation/MATLAB Function2 ==
  data: Vx input; V_FL output; Vy input; phi_dot input; delta_L input; V_FR output; V_RL output; V_RR output; alpha_FL output; alpha_FR output; alpha_RL output; alpha_RR output; delta_R input; a input; b input; t input; Vx_min input
function [V_FL,V_FR,V_RL,V_RR,alpha_FL,alpha_FR,alpha_RL,alpha_RR]= fcn(Vx,Vy,phi_dot, delta_L,delta_R,a,b,t,Vx_min)
   
    vx_max_den = max(Vx,Vx_min);

    V_FL = (Vx-(t/2)*phi_dot)*cos(delta_L)+(Vy+a*phi_dot)*sin(delta_L);
    alpha_FL = atan((Vy+a*phi_dot)/(vx_max_den -(t/2)*phi_dot))-delta_L;

    V_FR = (Vx+(t/2)*phi_dot)*cos(delta_R)+(Vy+a*phi_dot)*sin(delta_R);
    alpha_FR = atan((Vy+a*phi_dot)/(vx_max_den + (t/2)*phi_dot))-delta_R;

    V_RL = (((Vx-(t/2)*phi_dot)^2)+((Vy-b*phi_dot)^2))^(1/2);
    alpha_RL = atan((Vy-b*phi_dot)/(vx_max_den -(t/2)*phi_dot));

    V_RR = (((Vx+(t/2)*phi_dot)^2)+((Vy-b*phi_dot)^2))^(1/2);
    alpha_RR = atan((Vy-b*phi_dot)/(vx_max_den + (t/2)*phi_dot));
         
end

== stateflow chart TVModel/Subsystem/Subsystem1/Slip Control/Traction Control/Slip Control/TC/Activation logic ==
  state TS_ON
    state TC_OFF
      en:TC_Active=uint8(ones(4,1));
      en,du:
      T_max(1:4) = T_limit(1:4);
    state TC_ON
      state FL [parallel]
        settings: executionOrder=1
        state TC_ACTIVE
          en:
          TC_Active(1)=uint8(2);
          T_max(1) = abs(T_actual(1));
          du:
          T_max(1) = Tmax_PI(1);
        state TC_INACTIVE
          en:
          TC_Active(1)=uint8(1);
          T_max(1) = T_limit(1);
          du:
          T_max(1) = T_limit(1);
        (default) -> TS_ON.TC_ON.FL.TC_INACTIVE
        TS_ON.TC_ON.FL.TC_INACTIVE -> TS_ON.TC_ON.FL.TC_ACTIVE : [eps(1) >= epsTarget(1) + slipNoise]
        TS_ON.TC_ON.FL.TC_ACTIVE -> TS_ON.TC_ON.FL.TC_INACTIVE : [T_actual(1) < slipDeactPerc*Tmax_old(1)]
      state FR [parallel]
        settings: executionOrder=2
        state TC_ACTIVE
          en:
          TC_Active(2)=uint8(2);
          T_max(2) = abs(T_actual(2));
          du:
          T_max(2) = Tmax_PI(2);
        state TC_INACTIVE
          en:
          TC_Active(2)=uint8(1);
          T_max(2) = T_limit(2);
          du:
          T_max(2) = T_limit(2);
        (default) -> TS_ON.TC_ON.FR.TC_INACTIVE
        TS_ON.TC_ON.FR.TC_INACTIVE -> TS_ON.TC_ON.FR.TC_ACTIVE : [eps(2) >= epsTarget(2) + slipNoise]
        TS_ON.TC_ON.FR.TC_ACTIVE -> TS_ON.TC_ON.FR.TC_INACTIVE : [T_actual(2) < slipDeactPerc*Tmax_old(2) ]
      state RL [parallel]
        settings: executionOrder=3
        state TC_ACTIVE
          en:
          TC_Active(3)=uint8(2);
          T_max(3) = abs(T_actual(3));
          du:
          T_max(3) = Tmax_PI(3);
        state TC_INACTIVE
          en:
          TC_Active(3)=uint8(1);
          T_max(3) = T_limit(3);
          du:
          T_max(3) = T_limit(3);
        (default) -> TS_ON.TC_ON.RL.TC_INACTIVE
        TS_ON.TC_ON.RL.TC_INACTIVE -> TS_ON.TC_ON.RL.TC_ACTIVE : [eps(3) >= epsTarget(3) + slipNoise]
        TS_ON.TC_ON.RL.TC_ACTIVE -> TS_ON.TC_ON.RL.TC_INACTIVE : [T_actual(3) < slipDeactPerc*Tmax_old(3)]
      state RR [parallel]
        settings: executionOrder=4
        state TC_ACTIVE
          en:
          TC_Active(4)=uint8(2);
          T_max(4) = abs(T_actual(4));
          du:
          T_max(4) = Tmax_PI(4);
        state TC_INACTIVE
          en:
          TC_Active(4)=uint8(1);
          T_max(4) = T_limit(4);
          du:
          T_max(4) = T_limit(4);
        (default) -> TS_ON.TC_ON.RR.TC_INACTIVE
        TS_ON.TC_ON.RR.TC_INACTIVE -> TS_ON.TC_ON.RR.TC_ACTIVE : [eps(4) >= epsTarget(4) + slipNoise]
        TS_ON.TC_ON.RR.TC_ACTIVE -> TS_ON.TC_ON.RR.TC_INACTIVE : [T_actual(4) < slipDeactPerc*Tmax_old(4)]
    (default) -> TC_OFF
    TC_ON -> TC_OFF : [TC_flag == 0]
    TC_OFF -> TC_ON : [TC_flag == 1]
  state TS_OFF
    en:
    T_max(1:4) = zeros(4,1);
  (default) -> TS_OFF
  TS_OFF -> TS_ON : [RTD_flag == 1]
  TS_ON -> TS_OFF : [RTD_flag == 0]
  data: Tmax_PI input size=4; epsTarget input size=4; eps input size=4; T_actual input size=4 =zeros(4,1); T_max output size=4 =zeros(4,1); T_limit input size=4; TC_flag input size=1; Tmax_old input size=4; slipNoise input double =LV.slipNoise; slipDeactPerc input; RTD_flag input; TC_Active output uint8 size=4

== matlab function TVModel/Subsystem/Subsystem1/Slip Control/Traction Control/Slip Control/slip ratio/MATLAB Function ==
  data: vx_wheels input size=4; k output size=4; wR input size=4; vx_min input
function k = slipRatio(vx_wheels,wR,vx_min)

k = zeros(4,1);

for i = 1:4
   k(i) = (wR(i) - vx_wheels(i))/max([vx_wheels(i), wR(i), vx_min]);
end

end

== matlab function TVModel/Subsystem/Subsystem1/Torque Distribution/MPC/Mz Generation/MATLAB Function3 ==
  data: ubx input; lbx input; Mzlim output; delta input
function Mzlim = fcn(ubx,lbx,delta)
tf = 1.27;
tr = 1.27;
a = 0.765;

delta_l = delta(1);
delta_r = delta(2);

T_FL_max = ubx(1);
T_FR_min = lbx(2);
T_RL_max = ubx(3);
T_RR_min = lbx(4);

Mzlim = +(a.*sin(delta_l)-tf/2.*cos(delta_l))*T_FL_max +(a.*sin(delta_r)+tf/2*cos(delta_r))*T_FR_min -tr/2*T_RL_max +tr/2*T_RR_min;

== matlab function TVModel/Subsystem/Subsystem1/Torque Distribution/MPC/Mz Generation/MATLAB Function4 ==
  data: ubx input; lbx input; Mzlim output; delta input
function Mzlim = fcn(ubx,lbx,delta)
tf = 1.27;
tr = 1.27;
a = 0.765;

delta_l = delta(1);
delta_r = delta(2);

T_FL_min = lbx(1);
T_FR_max = ubx(2);
T_RL_min = lbx(3);
T_RR_max = ubx(4);

Mzlim = +(a.*sin(delta_l)-tf/2.*cos(delta_l))*T_FL_min +(a.*sin(delta_r)+tf/2*cos(delta_r))*T_FR_max -tr/2*T_RL_min +tr/2*T_RR_max;
